simulink model "cl_PD_bueno"  (R2024b)
settings: Solver=VariableStepAuto  StartTime=0.0  StopTime=Tmax  RelTol=1e-3
values from neighbouring files (symbols this model uses):
  Bm = [0.0014 0.0019 0.0022]    [controlled_robot_def_Nested.m]    (also in controlled_robot_def_PD.m; controlled_robot_def_PID.m; controlled_robot_def_ctorque.m; controlled_robot_def_freedfwrd.m)
  D = [2 9 5 5 5 5 5 8]    [Lagrangian_Method_3DOF_normal.m]    (also in circle_drawing.m; controlled_robot_def_PD.m = [Jm(1)/Bm(1) Jm(2)/Bm(2) Jm(3)/Bm(3)]; controlled_robot_def_PID.m = Td; robot_definition.m)
  Gear = [25 20 25]    [controlled_robot_def_Nested.m]    (also in controlled_robot_def_PD.m; controlled_robot_def_PID.m; controlled_robot_def_ctorque.m; controlled_robot_def_freedfwrd.m)
  Jm = [L(1).Jm L(2).Jm L(3).Jm]    [controlled_robot_def_Nested.m]    (also in controlled_robot_def_PD.m; controlled_robot_def_PID.m; controlled_robot_def_ctorque.m; controlled_robot_def_freedfwrd.m)
  km = [10 10 10]    [controlled_robot_def_Nested.m]    (also in controlled_robot_def_PD.m; controlled_robot_def_PID.m; controlled_robot_def_ctorque.m; controlled_robot_def_freedfwrd.m)
  N = [100 100 100]    [controlled_robot_def_Nested.m]    (also in controlled_robot_def_PD.m; controlled_robot_def_PID.m; controlled_robot_def_ctorque.m; controlled_robot_def_freedfwrd.m)
  P = [100*Bm(1)/km(1) 100*Bm(2)/km(2) 100*Bm(3)/km(3)]    [controlled_robot_def_PD.m]    (also in controlled_robot_def_PID.m = Kc)
  q_inicial = [0 0 0]    [circle_drawing.m]    (also in controlled_robot_def_Nested.m; controlled_robot_def_PD.m; controlled_robot_def_PID.m; controlled_robot_def_ctorque.m)
  qf = [pi/2 pi/8 pi/8]    [controlled_robot_def_Nested.m]    (also in controlled_robot_def_PD.m = [pi/2 pi/4 pi/4]; controlled_robot_def_PID.m; controlled_robot_def_ctorque.m; controlled_robot_def_freedfwrd.m)
  robot_3dof = SerialLink(L, 'name', 'Robot 3-DOF')    [circle_drawing.m]    (also in controlled_robot_def_Nested.m; controlled_robot_def_PD.m; controlled_robot_def_PID.m; controlled_robot_def_ctorque.m)
  Tm = Ts_calculated    [controlled_robot_def_Nested.m]    (also in controlled_robot_def_PD.m = 0.001; controlled_robot_def_PID.m; controlled_robot_def_ctorque.m; controlled_robot_def_freedfwrd.m)
  unc = 0.2    [controlled_robot_def_Nested.m]    (also in controlled_robot_def_PD.m; controlled_robot_def_PID.m = 0; controlled_robot_def_ctorque.m; controlled_robot_def_freedfwrd.m)
libraries: roblocks x5, slpidlib x4
settings Model: Creator=pcarn  LastModifiedBy=pablo

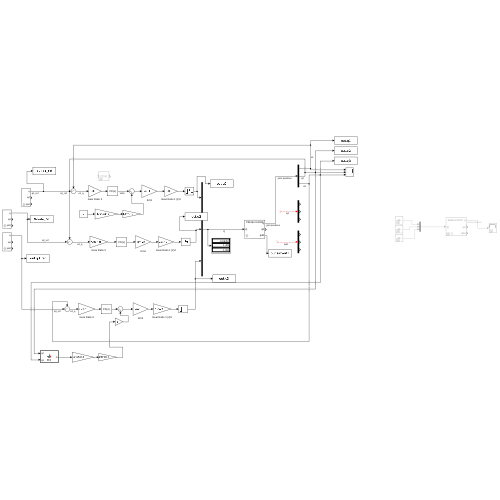
[thumbnail: Simulink's stored preview of the top-level diagram]
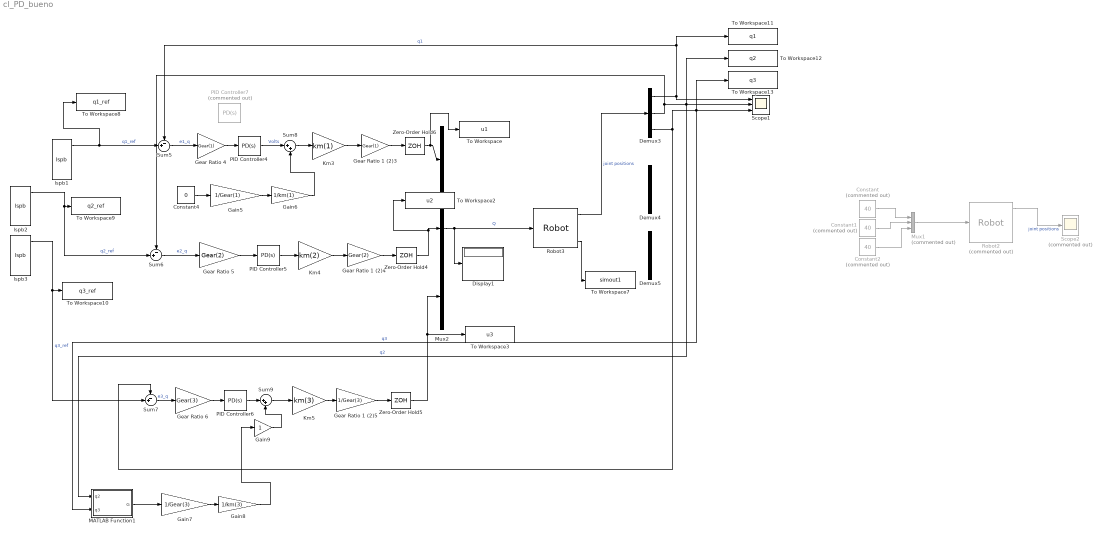
== system cl_PD_bueno ==
  Constant : Constant  Commented=on  Value=40
  Constant1 : Constant  Commented=on  Value=40
  Constant2 : Constant  Commented=on  Value=40
  Constant4 : Constant  Value=0
  Demux3 : Demux  Outputs=3
  Demux4 : Demux  Outputs=3
  Demux5 : Demux  Outputs=3
  Display1 : Display
  Gain5 : Gain  Gain=1/Gear(1)
  Gain6 : Gain  Gain=1/km(1)
  Gain7 : Gain  Gain=1/Gear(3)
  Gain8 : Gain  Gain=1/km(3)
  Gain9 : Gain
  Gear Ratio 1 (2)3 : Gain  Gain=Gear(1)
  Gear Ratio 1 (2)4 : Gain  Gain=Gear(2)
  Gear Ratio 1 (2)5 : Gain  Gain=1/Gear(3)
  Gear Ratio 4 : Gain  Gain=Gear(1)
  Gear Ratio 5 : Gain  Gain=Gear(2)
  Gear Ratio 6 : Gain  Gain=Gear(3)
  Km3 : Gain  Gain=km(1)
  Km4 : Gain  Gain=km(2)
  Km5 : Gain  Gain=km(3)
  MATLAB Function1 : MATLAB Function  TreatAsAtomicUnit=on
  Mux1 : Mux  Commented=on  Inputs=3
  Mux2 : Mux  Inputs=3
  PID Controller4 : slpidlib/PID Controller  Controller=PD  Form=Ideal  TimeDomain=Continuous-time  UseExternalTs=off  SampleTime=-1  IntegratorMethod=Forward Euler  FilterMethod=Forward Euler  ControllerParametersSource=internal  P=P(1)  I=1  UseKiTs=off  D=D(1)  UseExternalDerivativeSource=off  N=N(1)  UseFilter=on  TunerSelectOption=Transfer Function Based (PID Tuner App)  InitialConditionSource=internal  InitialConditionForIntegrator=0  InitialConditionForFilter=0  DifferentiatorICPrevScaledInput=0  ExternalReset=none  TrackingMode=off  Kt=1  LimitOutput=off  SatLimitsSource=internal  UpperSaturationLimit=inf  LowerSaturationLimit=-inf  LinearizeAsGain=on  AntiWindupMode=none  Kb=1  LimitIntegrator=off  UpperIntegratorSaturationLimit=inf  LowerIntegratorSaturationLimit=-inf  POutMin=[]  POutMax=[]  IOutMin=[]  IOutMax=[]  DOutMin=[]  DOutMax=[]  NOutMin=[]  NOutMax=[]  SumOutMin=[]  SumOutMax=[]  SaturationOutMin=[]  SaturationOutMax=[]  PParamMin=[]  PParamMax=[]  IParamMin=[]  IParamMax=[]  DParamMin=[]  DParamMax=[]  NParamMin=[]  NParamMax=[]  KbParamMin=[]  KbParamMax=[]  KtParamMin=[]  KtParamMax=[]  KbOutMin=[]  KbOutMax=[]  KtOutMin=[]  KtOutMax=[]  IntegratorOutMin=[]  IntegratorOutMax=[]  FilterOutMin=[]  FilterOutMax=[]  SumI1OutMin=[]  SumI1OutMax=[]  SumI2OutMin=[]  SumI2OutMax=[]  SumI3OutMin=[]  SumI3OutMax=[]  SumI4OutMin=[]  SumI4OutMax=[]  SumDOutMin=[]  SumDOutMax=[]  DifferentiatorOutMin=[]  DifferentiatorOutMax=[]  FilterDiffOutCoefMin=[]  FilterDiffOutCoefMax=[]  ReciprocalOutMin=[]  ReciprocalOutMax=[]  SumDenOutMin=[]  SumDenOutMax=[]  SumNumOutMin=[]  SumNumOutMax=[]  DivideOutMin=[]  DivideOutMax=[]  UdiffTsProdOutMin=[]  UdiffTsProdOutMax=[]  NTsProdOutMin=[]  NTsProdOutMax=[]  UintegralTsProdOutMin=[]  UintegralTsProdOutMax=[]  UngainTsProdOutMin=[]  UngainTsProdOutMax=[]  ClampingZeroOutDataTypeStr=Inherit: Inherit via back propagation  ClampingZeroOutMin=[]  ClampingZeroOutMax=[]  FilterDenConstantOutDataTypeStr=Inherit: Inherit via back propagation  FilterDenConstantOutMin=[]  FilterDenConstantOutMax=[]  PCopyOutDataTypeStr=Inherit: Inherit via back propagation  PCopyOutMin=[]  PCopyOutMax=[]  NCopyOutDataTypeStr=Inherit: Inherit via back propagation  NCopyOutMin=[]  NCopyOutMax=[]  IntegratorContinuousStateAttributes=''  IntegratorStateMustResolveToSignalObject=off  IntegratorRTWStateStorageClass=Auto  FilterContinuousStateAttributes=''  FilterStateMustResolveToSignalObject=off  FilterRTWStateStorageClass=Auto  ParallelPVariant=Passthrough  IdealPVariant=InternalParameters  IVariant=Disabled  DVariant=InternalParameters  IntegratorVariant=Disabled  SatVariant=Disabled  AWVariant=Disabled  PCopyVariant=Disabled  TRVariant=Disabled  FdbkBlocksVariant=Forward  IdealPFdbkVariant=Disabled  SatFdbkVariant=Disabled  DerivativeFilterVariant=ContFilter  NVariant=InternalParameters  NCopyVariant=Disabled  FilterICVariant=InternalICsFilter  IntegratorICVariant=Disabled  ExternalResetVariant=Disabled  TRSumVariant=Passthrough  SumFdbkVariant=Disabled  SumVariant=Sum_PD  TsampFilterVariant=InternalTs  TsampNgainVariant=Passthrough  TsampIntegralVariant=Disabled_SignalSpec  ExternalSaturationOutDataTypeStr=Inherit: Same as second input  DerivativeSourceVariant=ErrorSignal  PreIntVariant=InternalPreInt
  PID Controller5 : slpidlib/PID Controller  Controller=PD  Form=Ideal  TimeDomain=Continuous-time  UseExternalTs=off  SampleTime=-1  IntegratorMethod=Forward Euler  FilterMethod=Forward Euler  ControllerParametersSource=internal  P=P(2)  I=1  UseKiTs=off  D=D(2)  UseExternalDerivativeSource=off  N=N(2)  UseFilter=on  TunerSelectOption=Transfer Function Based (PID Tuner App)  InitialConditionSource=internal  InitialConditionForIntegrator=0  InitialConditionForFilter=0  DifferentiatorICPrevScaledInput=0  ExternalReset=none  TrackingMode=off  Kt=1  LimitOutput=off  SatLimitsSource=internal  UpperSaturationLimit=inf  LowerSaturationLimit=-inf  LinearizeAsGain=on  AntiWindupMode=none  Kb=1  LimitIntegrator=off  UpperIntegratorSaturationLimit=inf  LowerIntegratorSaturationLimit=-inf  POutMin=[]  POutMax=[]  IOutMin=[]  IOutMax=[]  DOutMin=[]  DOutMax=[]  NOutMin=[]  NOutMax=[]  SumOutMin=[]  SumOutMax=[]  SaturationOutMin=[]  SaturationOutMax=[]  PParamMin=[]  PParamMax=[]  IParamMin=[]  IParamMax=[]  DParamMin=[]  DParamMax=[]  NParamMin=[]  NParamMax=[]  KbParamMin=[]  KbParamMax=[]  KtParamMin=[]  KtParamMax=[]  KbOutMin=[]  KbOutMax=[]  KtOutMin=[]  KtOutMax=[]  IntegratorOutMin=[]  IntegratorOutMax=[]  FilterOutMin=[]  FilterOutMax=[]  SumI1OutMin=[]  SumI1OutMax=[]  SumI2OutMin=[]  SumI2OutMax=[]  SumI3OutMin=[]  SumI3OutMax=[]  SumI4OutMin=[]  SumI4OutMax=[]  SumDOutMin=[]  SumDOutMax=[]  DifferentiatorOutMin=[]  DifferentiatorOutMax=[]  FilterDiffOutCoefMin=[]  FilterDiffOutCoefMax=[]  ReciprocalOutMin=[]  ReciprocalOutMax=[]  SumDenOutMin=[]  SumDenOutMax=[]  SumNumOutMin=[]  SumNumOutMax=[]  DivideOutMin=[]  DivideOutMax=[]  UdiffTsProdOutMin=[]  UdiffTsProdOutMax=[]  NTsProdOutMin=[]  NTsProdOutMax=[]  UintegralTsProdOutMin=[]  UintegralTsProdOutMax=[]  UngainTsProdOutMin=[]  UngainTsProdOutMax=[]  ClampingZeroOutDataTypeStr=Inherit: Inherit via back propagation  ClampingZeroOutMin=[]  ClampingZeroOutMax=[]  FilterDenConstantOutDataTypeStr=Inherit: Inherit via back propagation  FilterDenConstantOutMin=[]  FilterDenConstantOutMax=[]  PCopyOutDataTypeStr=Inherit: Inherit via back propagation  PCopyOutMin=[]  PCopyOutMax=[]  NCopyOutDataTypeStr=Inherit: Inherit via back propagation  NCopyOutMin=[]  NCopyOutMax=[]  IntegratorContinuousStateAttributes=''  IntegratorStateMustResolveToSignalObject=off  IntegratorRTWStateStorageClass=Auto  FilterContinuousStateAttributes=''  FilterStateMustResolveToSignalObject=off  FilterRTWStateStorageClass=Auto  ParallelPVariant=Passthrough  IdealPVariant=InternalParameters  IVariant=Disabled  DVariant=InternalParameters  IntegratorVariant=Disabled  SatVariant=Disabled  AWVariant=Disabled  PCopyVariant=Disabled  TRVariant=Disabled  FdbkBlocksVariant=Forward  IdealPFdbkVariant=Disabled  SatFdbkVariant=Disabled  DerivativeFilterVariant=ContFilter  NVariant=InternalParameters  NCopyVariant=Disabled  FilterICVariant=InternalICsFilter  IntegratorICVariant=Disabled  ExternalResetVariant=Disabled  TRSumVariant=Passthrough  SumFdbkVariant=Disabled  SumVariant=Sum_PD  TsampFilterVariant=InternalTs  TsampNgainVariant=Passthrough  TsampIntegralVariant=Disabled_SignalSpec  ExternalSaturationOutDataTypeStr=Inherit: Same as second input  DerivativeSourceVariant=ErrorSignal  PreIntVariant=InternalPreInt
  PID Controller6 : slpidlib/PID Controller  Controller=PD  Form=Ideal  TimeDomain=Continuous-time  UseExternalTs=off  SampleTime=-1  IntegratorMethod=Forward Euler  FilterMethod=Forward Euler  ControllerParametersSource=internal  P=P(3)  I=1  UseKiTs=off  D=D(3)  UseExternalDerivativeSource=off  N=N(3)  UseFilter=on  TunerSelectOption=Transfer Function Based (PID Tuner App)  InitialConditionSource=internal  InitialConditionForIntegrator=0  InitialConditionForFilter=0  DifferentiatorICPrevScaledInput=0  ExternalReset=none  TrackingMode=off  Kt=1  LimitOutput=off  SatLimitsSource=internal  UpperSaturationLimit=inf  LowerSaturationLimit=-inf  LinearizeAsGain=on  AntiWindupMode=none  Kb=1  LimitIntegrator=off  UpperIntegratorSaturationLimit=inf  LowerIntegratorSaturationLimit=-inf  POutMin=[]  POutMax=[]  IOutMin=[]  IOutMax=[]  DOutMin=[]  DOutMax=[]  NOutMin=[]  NOutMax=[]  SumOutMin=[]  SumOutMax=[]  SaturationOutMin=[]  SaturationOutMax=[]  PParamMin=[]  PParamMax=[]  IParamMin=[]  IParamMax=[]  DParamMin=[]  DParamMax=[]  NParamMin=[]  NParamMax=[]  KbParamMin=[]  KbParamMax=[]  KtParamMin=[]  KtParamMax=[]  KbOutMin=[]  KbOutMax=[]  KtOutMin=[]  KtOutMax=[]  IntegratorOutMin=[]  IntegratorOutMax=[]  FilterOutMin=[]  FilterOutMax=[]  SumI1OutMin=[]  SumI1OutMax=[]  SumI2OutMin=[]  SumI2OutMax=[]  SumI3OutMin=[]  SumI3OutMax=[]  SumI4OutMin=[]  SumI4OutMax=[]  SumDOutMin=[]  SumDOutMax=[]  DifferentiatorOutMin=[]  DifferentiatorOutMax=[]  FilterDiffOutCoefMin=[]  FilterDiffOutCoefMax=[]  ReciprocalOutMin=[]  ReciprocalOutMax=[]  SumDenOutMin=[]  SumDenOutMax=[]  SumNumOutMin=[]  SumNumOutMax=[]  DivideOutMin=[]  DivideOutMax=[]  UdiffTsProdOutMin=[]  UdiffTsProdOutMax=[]  NTsProdOutMin=[]  NTsProdOutMax=[]  UintegralTsProdOutMin=[]  UintegralTsProdOutMax=[]  UngainTsProdOutMin=[]  UngainTsProdOutMax=[]  ClampingZeroOutDataTypeStr=Inherit: Inherit via back propagation  ClampingZeroOutMin=[]  ClampingZeroOutMax=[]  FilterDenConstantOutDataTypeStr=Inherit: Inherit via back propagation  FilterDenConstantOutMin=[]  FilterDenConstantOutMax=[]  PCopyOutDataTypeStr=Inherit: Inherit via back propagation  PCopyOutMin=[]  PCopyOutMax=[]  NCopyOutDataTypeStr=Inherit: Inherit via back propagation  NCopyOutMin=[]  NCopyOutMax=[]  IntegratorContinuousStateAttributes=''  IntegratorStateMustResolveToSignalObject=off  IntegratorRTWStateStorageClass=Auto  FilterContinuousStateAttributes=''  FilterStateMustResolveToSignalObject=off  FilterRTWStateStorageClass=Auto  ParallelPVariant=Passthrough  IdealPVariant=InternalParameters  IVariant=Disabled  DVariant=InternalParameters  IntegratorVariant=Disabled  SatVariant=Disabled  AWVariant=Disabled  PCopyVariant=Disabled  TRVariant=Disabled  FdbkBlocksVariant=Forward  IdealPFdbkVariant=Disabled  SatFdbkVariant=Disabled  DerivativeFilterVariant=ContFilter  NVariant=InternalParameters  NCopyVariant=Disabled  FilterICVariant=InternalICsFilter  IntegratorICVariant=Disabled  ExternalResetVariant=Disabled  TRSumVariant=Passthrough  SumFdbkVariant=Disabled  SumVariant=Sum_PD  TsampFilterVariant=InternalTs  TsampNgainVariant=Passthrough  TsampIntegralVariant=Disabled_SignalSpec  ExternalSaturationOutDataTypeStr=Inherit: Same as second input  DerivativeSourceVariant=ErrorSignal  PreIntVariant=InternalPreInt
  PID Controller7 : slpidlib/PID Controller  Commented=on  Controller=PD  Form=Ideal  TimeDomain=Continuous-time  UseExternalTs=off  SampleTime=-1  IntegratorMethod=Forward Euler  FilterMethod=Forward Euler  ControllerParametersSource=internal  P=Jm(1)/Bm(1)  I=1  UseKiTs=off  D=100*Bm(1)/km(1)  UseExternalDerivativeSource=off  N=N(1)  UseFilter=on  TunerSelectOption=Transfer Function Based (PID Tuner App)  InitialConditionSource=internal  InitialConditionForIntegrator=0  InitialConditionForFilter=0  DifferentiatorICPrevScaledInput=0  ExternalReset=none  TrackingMode=off  Kt=1  LimitOutput=off  SatLimitsSource=internal  UpperSaturationLimit=inf  LowerSaturationLimit=-inf  LinearizeAsGain=on  AntiWindupMode=none  Kb=1  LimitIntegrator=off  UpperIntegratorSaturationLimit=inf  LowerIntegratorSaturationLimit=-inf  POutMin=[]  POutMax=[]  IOutMin=[]  IOutMax=[]  DOutMin=[]  DOutMax=[]  NOutMin=[]  NOutMax=[]  SumOutMin=[]  SumOutMax=[]  SaturationOutMin=[]  SaturationOutMax=[]  PParamMin=[]  PParamMax=[]  IParamMin=[]  IParamMax=[]  DParamMin=[]  DParamMax=[]  NParamMin=[]  NParamMax=[]  KbParamMin=[]  KbParamMax=[]  KtParamMin=[]  KtParamMax=[]  KbOutMin=[]  KbOutMax=[]  KtOutMin=[]  KtOutMax=[]  IntegratorOutMin=[]  IntegratorOutMax=[]  FilterOutMin=[]  FilterOutMax=[]  SumI1OutMin=[]  SumI1OutMax=[]  SumI2OutMin=[]  SumI2OutMax=[]  SumI3OutMin=[]  SumI3OutMax=[]  SumI4OutMin=[]  SumI4OutMax=[]  SumDOutMin=[]  SumDOutMax=[]  DifferentiatorOutMin=[]  DifferentiatorOutMax=[]  FilterDiffOutCoefMin=[]  FilterDiffOutCoefMax=[]  ReciprocalOutMin=[]  ReciprocalOutMax=[]  SumDenOutMin=[]  SumDenOutMax=[]  SumNumOutMin=[]  SumNumOutMax=[]  DivideOutMin=[]  DivideOutMax=[]  UdiffTsProdOutMin=[]  UdiffTsProdOutMax=[]  NTsProdOutMin=[]  NTsProdOutMax=[]  UintegralTsProdOutMin=[]  UintegralTsProdOutMax=[]  UngainTsProdOutMin=[]  UngainTsProdOutMax=[]  ClampingZeroOutDataTypeStr=Inherit: Inherit via back propagation  ClampingZeroOutMin=[]  ClampingZeroOutMax=[]  FilterDenConstantOutDataTypeStr=Inherit: Inherit via back propagation  FilterDenConstantOutMin=[]  FilterDenConstantOutMax=[]  PCopyOutDataTypeStr=Inherit: Inherit via back propagation  PCopyOutMin=[]  PCopyOutMax=[]  NCopyOutDataTypeStr=Inherit: Inherit via back propagation  NCopyOutMin=[]  NCopyOutMax=[]  IntegratorContinuousStateAttributes=''  IntegratorStateMustResolveToSignalObject=off  IntegratorRTWStateStorageClass=Auto  FilterContinuousStateAttributes=''  FilterStateMustResolveToSignalObject=off  FilterRTWStateStorageClass=Auto  ParallelPVariant=Passthrough  IdealPVariant=InternalParameters  IVariant=Disabled  DVariant=InternalParameters  IntegratorVariant=Disabled  SatVariant=Disabled  AWVariant=Disabled  PCopyVariant=Disabled  TRVariant=Disabled  FdbkBlocksVariant=Forward  IdealPFdbkVariant=Disabled  SatFdbkVariant=Disabled  DerivativeFilterVariant=ContFilter  NVariant=InternalParameters  NCopyVariant=Disabled  FilterICVariant=InternalICsFilter  IntegratorICVariant=Disabled  ExternalResetVariant=Disabled  TRSumVariant=Passthrough  SumFdbkVariant=Disabled  SumVariant=Sum_PD  TsampFilterVariant=InternalTs  TsampNgainVariant=Passthrough  TsampIntegralVariant=Disabled_SignalSpec  ExternalSaturationOutDataTypeStr=Inherit: Same as second input  DerivativeSourceVariant=ErrorSignal  PreIntVariant=InternalPreInt
  Robot2 : roblocks/Arm/Robot  Commented=on  robot=robot_3dof  q0=q_inicial
  Robot3 : roblocks/Arm/Robot  robot=robot_3dof.perturb(unc)  q0=q_inicial
  Scope1 : Scope  NumInputPorts=3
  Scope2 : Scope  Commented=on
  Sum5 : Sum  Inputs=-+|
  Sum6 : Sum  Inputs=-+|
  Sum7 : Sum  Inputs=-+|
  Sum8 : Sum  Inputs=|++
  Sum9 : Sum  Inputs=|++
  To Workspace : ToWorkspace  VariableName=u1  SaveFormat=Timeseries  SampleTime=-1
  To Workspace10 : ToWorkspace  VariableName=q3_ref  SaveFormat=Timeseries  SampleTime=-1
  To Workspace11 : ToWorkspace  VariableName=q1  SaveFormat=Timeseries  SampleTime=-1
  To Workspace12 : ToWorkspace  VariableName=q2  SaveFormat=Timeseries  SampleTime=-1
  To Workspace13 : ToWorkspace  VariableName=q3  SaveFormat=Timeseries  SampleTime=-1
  To Workspace2 : ToWorkspace  VariableName=u2  SaveFormat=Timeseries  SampleTime=-1
  To Workspace3 : ToWorkspace  VariableName=u3  SaveFormat=Timeseries  SampleTime=-1
  To Workspace7 : ToWorkspace  VariableName=simout1  SaveFormat=Timeseries  SampleTime=-1
  To Workspace8 : ToWorkspace  VariableName=q1_ref  SaveFormat=Timeseries  SampleTime=-1
  To Workspace9 : ToWorkspace  VariableName=q2_ref  SaveFormat=Timeseries  SampleTime=-1
  Zero-Order Hold4 : ZeroOrderHold  SampleTime=Tm
  Zero-Order Hold5 : ZeroOrderHold  SampleTime=Tm
  Zero-Order Hold6 : ZeroOrderHold  SampleTime=Tm
  lspb1 : roblocks/Toolbox/lspb  q0=q_inicial(1)  qf=qf(1)  tmax=Tmax
  lspb2 : roblocks/Toolbox/lspb  q0=q_inicial(2)  qf=qf(2)  tmax=Tmax
  lspb3 : roblocks/Toolbox/lspb  q0=q_inicial(3)  qf=qf(3)  tmax=Tmax
  wires:
  Mux1/1 -> Robot2/1
  Robot2/1 -> Scope2/1  "joint positions"
  Constant2/1 -> Mux1/3
  Constant1/1 -> Mux1/2
  Constant/1 -> Mux1/1
  Gain6/1 -> Sum8/2
  Gear Ratio 5/1 -> PID Controller5/1
  Sum9/1 -> Km5/1
  PID Controller6/1 -> Sum9/1
  Zero-Order Hold6/1 -> To Workspace/1, Mux2/1
  Km5/1 -> Gear Ratio 1 (2)5/1
  ? -> Demux5/1  "qdd"
  lspb1/1 -> To Workspace8/1, Sum5/2  "q1_ref"
  Gear Ratio 1 (2)4/1 -> Zero-Order Hold4/1
  Zero-Order Hold5/1 -> To Workspace3/1, Mux2/3
  Sum8/1 -> Km3/1
  Km3/1 -> Gear Ratio 1 (2)3/1
  MATLAB Function1/1(G) -> Gain7/1
  Demux3/2 -> Sum6/1, Scope1/2, To Workspace12/1, MATLAB Function1/1(q2)  "q2"
  PID Controller5/1 -> Km4/1
  Demux3/1 -> To Workspace11/1, Sum5/1, Scope1/1  "q1"
  Sum5/1 -> Gear Ratio 4/1  "e1_q"
  Gear Ratio 1 (2)5/1 -> Zero-Order Hold5/1
  Gain7/1 -> Gain8/1
  Mux2/1 -> Display1/1, Robot3/1  "Q"
  Constant4/1 -> Gain5/1
  Demux3/3 -> To Workspace13/1, MATLAB Function1/2(q3), Scope1/3, Sum7/1  "q3"
  Sum6/1 -> Gear Ratio 5/1  "e2_q"
  Gain8/1 -> Gain9/1
  lspb3/1 -> Sum7/2, To Workspace10/1  "q3_ref"
  Gear Ratio 4/1 -> PID Controller4/1
  Robot3/3 -> To Workspace7/1
  Robot3/1 -> Demux3/1  "joint positions"
  Gain5/1 -> Gain6/1
  PID Controller4/1 -> Sum8/1  "Volts"
  Gear Ratio 6/1 -> PID Controller6/1
  Sum7/1 -> Gear Ratio 6/1  "e3_q"
  Km4/1 -> Gear Ratio 1 (2)4/1
  ? -> Demux4/1  "qd"
  Gear Ratio 1 (2)3/1 -> Zero-Order Hold6/1
  Gain9/1 -> Sum9/2
  Zero-Order Hold4/1 -> To Workspace2/1, Mux2/2
  lspb2/1 -> Sum6/2, To Workspace9/1  "q2_ref"

== matlab function cl_PD_bueno/MATLAB Function1 ==
  data: q2 input; G output; q3 input
function G = fcn(q2, q3)
    
    D = [2 9 5 5 5 5 5 8];

    L1a_val = 0.9 - 0.04*D(2); 
    L2a_val = 0.4 + 0.02*D(6); 
    L3a_val = 0.4 + 0.01*D(3); 
    L4a_val = 0.5 - 0.02*D(7);
    
    m1_val = 4;
    m2_val = 2.7;
    m3_val = 2;

    
G = 9.81*L4a_val*m3_val*cos(q2+q3);
